simulink model "lab1_4"  (R2022a)
settings: Solver=VariableStepAuto  StartTime=0.0  StopTime=10.0  RelTol=1e-3
settings Model: Creator=Paulo  LastModifiedBy=Paulo

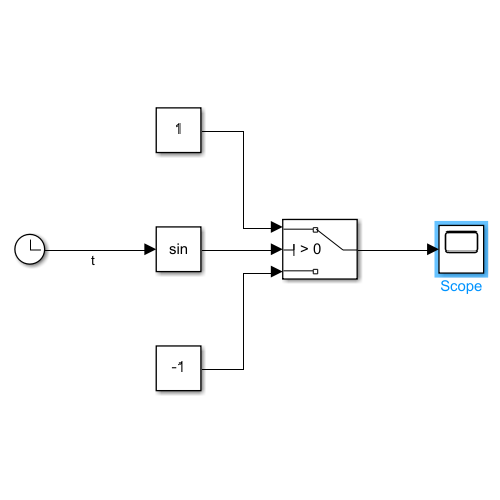
[thumbnail: Simulink's stored preview of the top-level diagram]
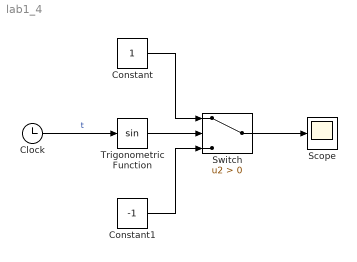
== system lab1_4 ==
  Clock : Clock
  Constant : Constant
  Constant1 : Constant  Value=-1
  Scope : Scope
  Switch : Switch  Criteria=u2 > Threshold  SaturateOnIntegerOverflow=off  InputSameDT=off
  Trigonometric Function : Trigonometry
  wires:
  Trigonometric Function/1 -> Switch/2
  Constant1/1 -> Switch/3
  Constant/1 -> Switch/1
  Clock/1 -> Trigonometric Function/1  "t"
  Switch/1 -> Scope/1
